simulink model "Basic_IO"  (R2021a)
settings: Solver=ode2  StartTime=0.0  StopTime=inf  FixedStep=0.002  RelTol=1e-3  EnableMultiTasking=on
undefined symbols (not defined in the file): HIL
libraries: quarc_library x9, simulink x2
settings Model: SimulationMode=external  ExtModeTrigDuration=10000  Creator=mbohra  LastModifiedBy=User
settings SolverCC: AlgebraicLoopSolver=TrustRegion  PositivePriorityOrder=on
settings DataIOCC: SaveOutput=off  SignalLogging=off  DSMLogging=off  SaveTime=off  ReturnWorkspaceOutputs=off
settings DebuggingCC: SFMachineParentedDataDiag=warning  ArithmeticOperatorsInVariantConditions=warning
settings HardwareCC: ProdBitPerLong=64  ProdLargestAtomicInteger=LongLong  ProdLargestAtomicFloat=Double  ProdLongLongMode=on  ProdHWDeviceType=ARM Compatible->ARM 64-bit (LP64)
settings SFSimCC: CustomCodeUndefinedFunction=UseInterfaceOnly
settings RTWCC: Description=QUARC Linux Nvidia Target (QCar) Using Toolchain  SystemTargetFile=quarc_linux_nvidia.tlc  TemplateMakefile=quarc_default_tmf  Toolchain=QUARC linux_nvidia | gmake (64-bit Windows)  BuildConfiguration=Faster Runs
settings STFCustomTargetCC: TargetLangStandard=C99 (ISO)  ConcurrentExecutionCompliant=on  SystemTargetFile=quarc_linux_nvidia.tlc
settings GRTTargetCC: ParMdlRefBuildCompliant=off  CompOptLevelCompliant=off  CombineOutputUpdateFcns=off  MatFileLogging=off  CPPClassGenCompliant=off  GRTInterface=on  ExtMode=on  ExtModeMexFile=quarc_comm  ExtModeMexArgs='-w -d /tmp -uri %u','tcpip://192.168.2.12:17001'

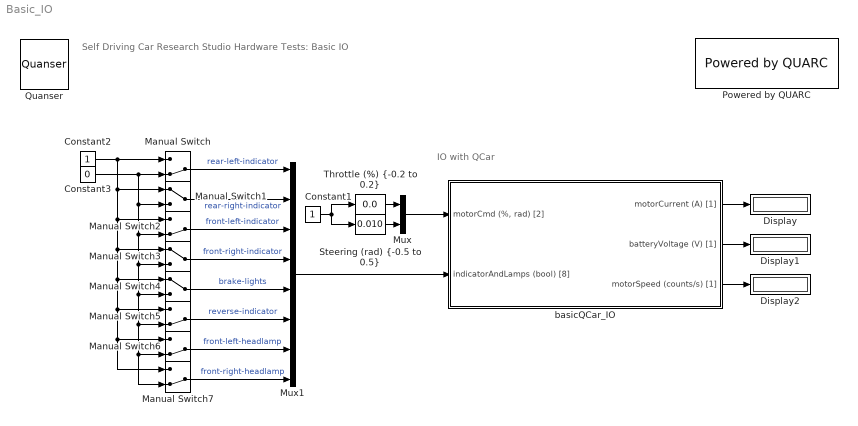
== system Basic_IO ==
  note: IO with QCar
  note: Self Driving Car Research Studio
      | Hardware Tests: Basic IO
  Constant1 : Constant
  Constant2 : Constant
  Constant3 : Constant  Value=0
  Display : Display
      settings: Decimation=0.5/qc_get_step_size
  Display1 : Display
      settings: Decimation=0.5/qc_get_step_size
  Display2 : Display
      settings: Decimation=0.5/qc_get_step_size
  Manual Switch{,2,5..7} (5 alike) : ManualSwitch  CurrentSetting=0
  Manual Switch1 : ManualSwitch
  Manual Switch3 : ManualSwitch
  Manual Switch4 : ManualSwitch
  Mux : Mux  Inputs=2
  Mux1 : Mux  Inputs=8
  Powered by QUARC : quarc_library/Logos/Powered by QUARC
  Quanser : quarc_library/Logos/Quanser
  "Steering (rad) {-0.5 to 0.5}" : simulink/Math Operations/Slider Gain  gain=0.010  low=-0.5  high=0.5
  "Throttle (%) {-0.2 to 0.2}" : simulink/Math Operations/Slider Gain  gain=0.0  low=-0.1  high=0.1
  basicQCar_IO : Subsystem
  wires:
  basicQCar_IO/3(motorSpeed (counts/s) [1]) -> Display2/1
  basicQCar_IO/2(batteryVoltage (V) [1]) -> Display1/1
  basicQCar_IO/1(motorCurrent (A) [1]) -> Display/1
  Mux1/1 -> basicQCar_IO/2(indicatorAndLamps (bool) [8])
  Mux/1 -> basicQCar_IO/1("motorCmd (%, rad) [2]")
  Constant1/1 -> "Throttle (%) {-0.2 to 0.2}"/1, "Steering (rad) {-0.5 to 0.5}"/1
  "Steering (rad) {-0.5 to 0.5}"/1 -> Mux/2
  "Throttle (%) {-0.2 to 0.2}"/1 -> Mux/1
  Constant3/1 -> Manual Switch4/2, Manual Switch5/2, Manual Switch6/2, Manual Switch7/2, Manual Switch3/2, Manual Switch2/2, Manual Switch1/2, Manual Switch/2
  Constant2/1 -> Manual Switch4/1, Manual Switch5/1, Manual Switch6/1, Manual Switch7/1, Manual Switch3/1, Manual Switch2/1, Manual Switch1/1, Manual Switch/1
  Manual Switch/1 -> Mux1/1  "rear-left-indicator"
  Manual Switch1/1 -> Mux1/2  "rear-right-indicator"
  Manual Switch2/1 -> Mux1/3  "front-left-indicator"
  Manual Switch3/1 -> Mux1/4  "front-right-indicator"
  Manual Switch4/1 -> Mux1/5  "brake-lights"
  Manual Switch5/1 -> Mux1/6  "reverse-indicator"
  Manual Switch6/1 -> Mux1/7  "front-left-headlamp"
  Manual Switch7/1 -> Mux1/8  "front-right-headlamp"

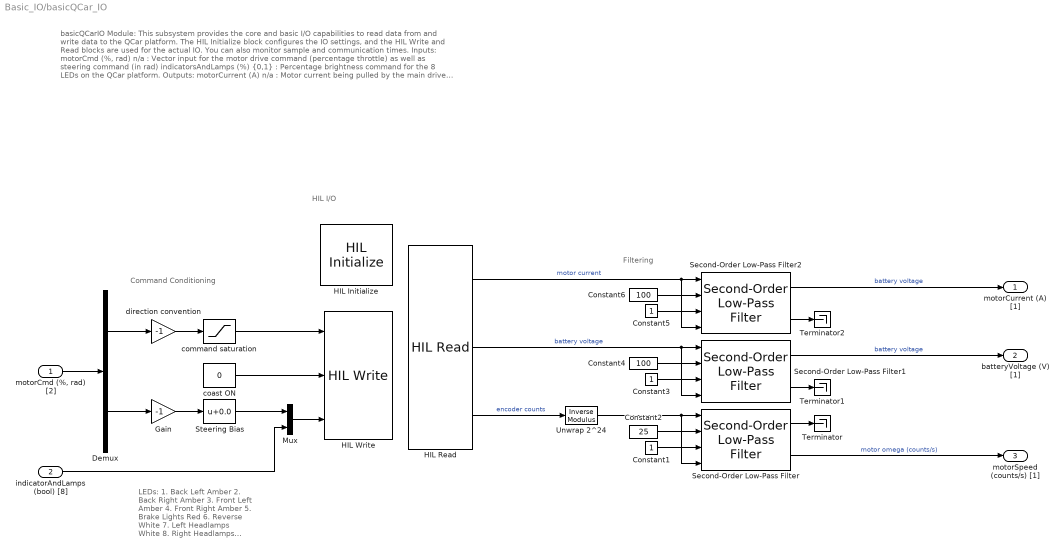
== system Basic_IO/basicQCar_IO ==
  note: Filtering
  note: basicQCarIO Module:
      |
      | This subsystem provides the core and basic I/O capabilities to read data from and write data to the QCar platform. The HIL Initialize block configures the IO settings, and the HIL Write and Read blocks are used for the actual IO. You can also monitor sample and communication times.
      |
      | Inputs:
      | motorCmd (%, rad) n/a : Vector input for the motor drive command (percentage throttle) as well as steering command (in rad)
      | indicatorsAndLamps (%) {0,1} : Percentage brightness command for the 8 LEDs on the QCar platform.
      |
      | Outputs:
      | motorCurrent (A) n/a : Motor current being pulled by the main drive motor
      | batteryVoltage (V) {0, 12.6} : Current battery voltage reading
      | motorSpeed (counts/s) n/a : Drive motor speed measured using an encoder (do not confuse with wheel speed as this measurement is at the drive shaft)
  note: Command Conditioning
  note: HIL I/O
  note: LEDs:
      | 1. Back Left Amber
      | 2. Back Right Amber
      | 3. Front Left Amber
      | 4. Front Right Amber
      | 5. Brake Lights Red
      | 6. Reverse White
      | 7. Left Headlamps White
      | 8. Right Headlamps White
  "motorCmd (%, rad) [2]" : Inport
  indicatorAndLamps (bool) [8] : Inport  Port=2
  Constant1 : Constant
  Constant2 : Constant  Value=25
  Constant3 : Constant
  Constant4 : Constant  Value=100
  Constant5 : Constant
  Constant6 : Constant  Value=100
  Demux : Demux  Outputs=2
  Gain : Gain  Gain=-1
  HIL Initialize : quarc_library/Data Acquisition/Generic/Configuration/HIL Initialize  object_name=HIL-1  board_type=qcar  board_number=0  board_options=""  exclusive=off  active=on  hardware_clocks=[]  clock_modes=[]  initial_clock_frequencies=[]  set_clock_params_at_start=off  set_clock_params_at_switch_in=off  set_clock_frequencies_at_start=off  set_clock_frequencies_at_switch_in=off  analog_input_channels=[0:6]  analog_input_configurations=[]  analog_input_maximums=[3.3]  analog_input_minimums=[0]  set_analog_input_params_at_start=off  set_analog_input_params_at_switch_in=off  analog_output_channels=[]  analog_output_maximums=[]  analog_output_minimums=[]  initial_analog_outputs=[]  final_analog_outputs=[]  watchdog_analog_outputs=[]  set_analog_output_params_at_start=off  set_analog_output_params_at_switch_in=off  set_analog_outputs_at_start=off  set_analog_outputs_at_switch_in=off  set_analog_outputs_at_terminate=off  set_analog_outputs_at_switch_out=off  set_analog_outputs_on_watchdog=off  digital_input_channels=[24:42]  digital_output_channels=[40]  digital_output_configuration=[]  initial_digital_outputs=[0]  final_digital_outputs=[1]  watchdog_digital_outputs=[]  set_digital_output_params_at_start=off  set_digital_output_params_at_switch_in=off  set_digital_outputs_at_start=on  set_digital_outputs_at_switch_in=off  set_digital_outputs_at_terminate=on  set_digital_outputs_at_switch_out=off  set_digital_outputs_on_watchdog=off  encoder_channels=[0:4]  quadrature=[4 4]  encoder_filter_frequency=100e6/1  initial_encoder_counts=[0]  set_encoder_params_at_start=on  set_encoder_params_at_switch_in=off  set_encoder_counts_at_start=on  set_encoder_counts_at_switch_in=off  pwm_channels=[0]  pwm_modes=[0 0]  pwm_frequency=150e6/4096  pwm_configuration=[0]  pwm_alignment=[0]  pwm_polarity=[1]  pwm_leading_deadband=[]  pwm_trailing_deadband=[]  initial_pwm_outputs=[0]  final_pwm_outputs=[0]  watchdog_pwm_outputs=[0]  set_pwm_params_at_start=on  set_pwm_params_at_switch_in=off  set_pwm_outputs_at_start=on  set_pwm_outputs_at_switch_in=off  set_pwm_outputs_at_terminate=on  set_pwm_outputs_at_switch_out=off  set_pwm_outputs_on_watchdog=off  other_output_channels=[1000, 11000:11011]  initial_other_outputs=[0]  final_other_outputs=[0]  watchdog_other_outputs=[]  set_other_outputs_at_start=on  set_other_outputs_at_switch_in=off  set_other_outputs_at_terminate=on  set_other_outputs_at_switch_out=off  set_other_outputs_on_watchdog=off
  HIL Read : quarc_library/Data Acquisition/Generic/Immediate I//O/HIL Read  object_name=HIL-1  analog_channels=[5:6]  encoder_channels=[0]  digital_channels=[]  other_channels=[]  sample_time=qc_get_step_size  active=on  vector_output=off  data_type_mode=Inherit via back propagation  encoder_data_type=double  digital_data_type=boolean
  HIL Write : quarc_library/Data Acquisition/Generic/Immediate I//O/HIL Write  object_name=HIL-1  analog_channels=[]  pwm_channels=[0]  digital_channels=[40]  other_channels=[1000 11008:11011 11000:11003]  sample_time=-1  active=off  vector_input=on
  Mux : Mux  Inputs=2
  Second-Order Low-Pass Filter : quarc_library/Continuous/Second-Order Low-Pass Filter  params_source=External (input ports)  input_width=1  input_zeta=1  input_init=0
  Second-Order Low-Pass Filter1 : quarc_library/Continuous/Second-Order Low-Pass Filter  params_source=External (input ports)  input_width=1  input_zeta=1  input_init=0
  Second-Order Low-Pass Filter2 : quarc_library/Continuous/Second-Order Low-Pass Filter  params_source=External (input ports)  input_width=1  input_zeta=1  input_init=0
  Steering Bias : Bias  Bias=0.0
  Terminator : Terminator
  Terminator1 : Terminator
  Terminator2 : Terminator
  Unwrap 2^24 : quarc_library/Discontinuities/Inverse Modulus  modulus=16777215  output_derivative=off  output_revolutions=off  max_x=Inf  min_x=-Inf
  coast ON : Constant  Value=0
  command saturation : Saturate  UpperLimit=0.20  LowerLimit=-0.20
  direction convention : Gain  Gain=-1
  motorCurrent (A) [1] : Outport  VectorParamsAs1DForOutWhenUnconnected=off
  batteryVoltage (V) [1] : Outport  Port=2  VectorParamsAs1DForOutWhenUnconnected=off
  motorSpeed (counts/s) [1] : Outport  Port=3  VectorParamsAs1DForOutWhenUnconnected=off
  wires:
  Second-Order Low-Pass Filter2/1 -> motorCurrent (A) [1]/1  "battery voltage"
  Constant2/1 -> Second-Order Low-Pass Filter/2
  Unwrap 2^24/1 -> Second-Order Low-Pass Filter/1, Second-Order Low-Pass Filter/4
  Demux/2 -> Gain/1
  direction convention/1 -> command saturation/1
  "motorCmd (%, rad) [2]"/1 -> Demux/1
  command saturation/1 -> HIL Write/1
  coast ON/1 -> HIL Write/2
  Second-Order Low-Pass Filter/1 -> Terminator/1
  Constant3/1 -> Second-Order Low-Pass Filter1/3
  indicatorAndLamps (bool) [8]/1 -> Mux/2
  Steering Bias/1 -> Mux/1
  Second-Order Low-Pass Filter1/1 -> batteryVoltage (V) [1]/1  "battery voltage"
  Constant5/1 -> Second-Order Low-Pass Filter2/3
  Second-Order Low-Pass Filter1/2 -> Terminator1/1
  HIL Read/2 -> Second-Order Low-Pass Filter1/1, Second-Order Low-Pass Filter1/4  "battery voltage"
  Mux/1 -> HIL Write/3
  Constant6/1 -> Second-Order Low-Pass Filter2/2
  Second-Order Low-Pass Filter/2 -> motorSpeed (counts/s) [1]/1  "motor omega (counts/s)"
  Second-Order Low-Pass Filter2/2 -> Terminator2/1
  Constant4/1 -> Second-Order Low-Pass Filter1/2
  Constant1/1 -> Second-Order Low-Pass Filter/3
  Demux/1 -> direction convention/1
  HIL Read/3 -> Unwrap 2^24/1  "encoder counts"
  HIL Read/1 -> Second-Order Low-Pass Filter2/1, Second-Order Low-Pass Filter2/4  "motor current"
  Gain/1 -> Steering Bias/1
